simulink model "AutomatedVehicle"  (R2024a)
settings: Solver=FixedStepAuto  StartTime=0.0  StopTime=Tend  FixedStep=Ts  RelTol=1e-3
values from neighbouring files (symbols this model uses):
  ego_v = [4.98933333333 4.97866666667 4.968 4.95733333333 4.94666666667 4.936 4.92533333333 4.91466666667 4.904 4.89333333333 4.88266666667 4.872 ... (5799 elements, 5799x1)]    [SimulationData.mat]    (also in get_Data.m = [ego_v; v])
  ego_x = [2.54994666667 2.59978666667 2.64952 2.69914666667 2.74866666667 2.79808 2.84738666667 2.89658666667 2.94568 2.99466666667 3.04354666667 3.09232 ... (5799 elements, 5799x1)]    [SimulationData.mat]    (also in get_Data.m = [ego_x; egoVehicle.Position(1)])
  ego_y = [-1.65 -1.65 -1.65 -1.65 -1.65 -1.65 -1.65 -1.65 -1.65 -1.65 -1.65 -1.65 ... (5799 elements, 5799x1)]    [SimulationData.mat]    (also in get_Data.m = [ego_y; egoVehicle.Position(2)])
  ego_yaw = [0 0 0 0 0 0 0 0 0 0 0 0 ... (5799 elements, 5799x1)]    [SimulationData.mat]    (also in get_Data.m = [ego_yaw; yaw])
  K1 = Kvec{1}    [Main.m]
  K2 = Kvec{2}    [Main.m]
  K3 = Kvec{3}    [Main.m]
  K4 = Kvec{4}    [Main.m]
  K5 = Kvec{5}    [Main.m]
  K6 = Kvec{6}    [Main.m]
  L = 2.8    [Main.m]
  tau = 0.5    [Main.m]
libraries: simulink x1
settings Model: Creator=mirko  LastModifiedBy=giuco
settings SolverCC: AlgebraicLoopSolver=TrustRegion
settings OptimizationCC: ReuseModelBlockBuffer=off
settings DebuggingCC: UnconnectedInputMsg=warning  UnconnectedOutputMsg=warning  UnconnectedLineMsg=warning
settings ModelReferenceCC: EnableRefExpFcnMdlSchedulingChecks=on
settings SFSimCC: CustomCodeUndefinedFunction=UseInterfaceOnly
settings RTWCC: GPUComputeCapability=3.5

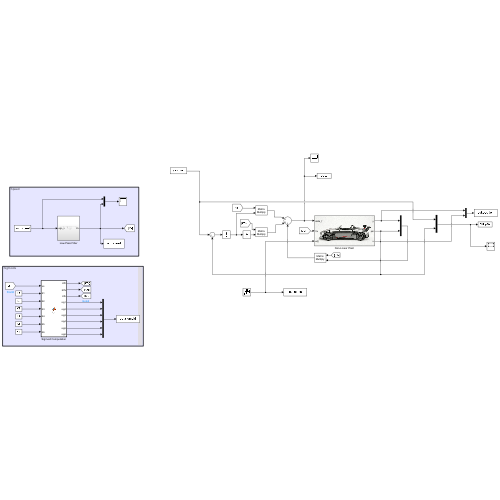
[thumbnail: Simulink's stored preview of the top-level diagram]
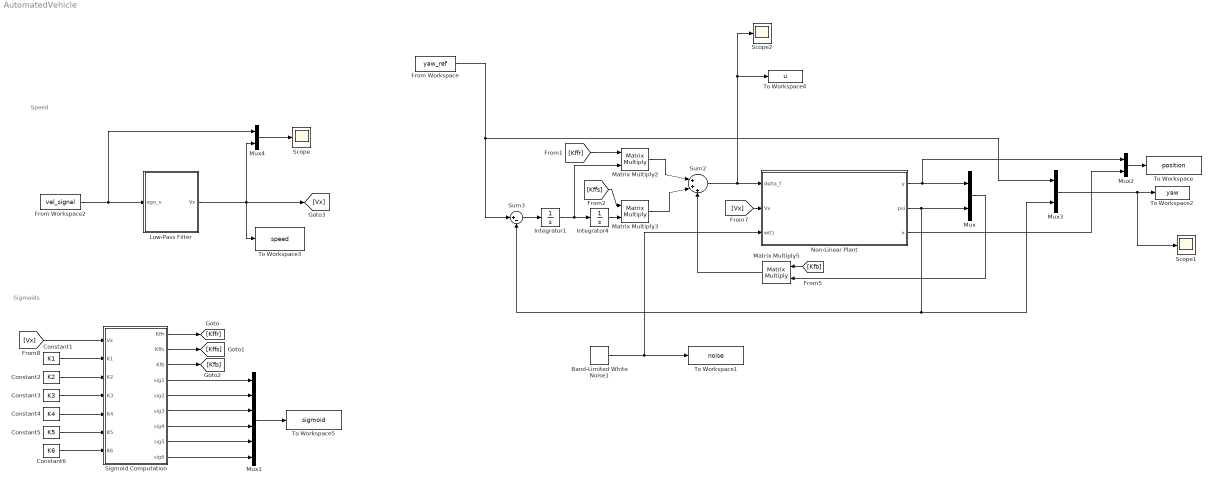
== system AutomatedVehicle ==
  note: Sigmoids
  note: Speed
  Band-Limited White Noise1 : simulink/Sources/Band-Limited White Noise  Cov=[0.001]  Ts=0.1  seed=[23341]
  Constant1 : Constant  Value=K1  VectorParams1D=off
  Constant2 : Constant  Value=K2  VectorParams1D=off
  Constant3 : Constant  Value=K3  VectorParams1D=off
  Constant4 : Constant  Value=K4  VectorParams1D=off
  Constant5 : Constant  Value=K5  VectorParams1D=off
  Constant6 : Constant  Value=K6  VectorParams1D=off
  From Workspace : FromWorkspace  VariableName=yaw_ref
  From Workspace2 : FromWorkspace  VariableName=vel_signal
  Integrator1 : Integrator
  Integrator4 : Integrator
  Low-Pass Filter : Subsystem
  Matrix Multiply2 : Product  Multiplication=Matrix(*)
  Matrix Multiply3 : Product  Multiplication=Matrix(*)
  Matrix Multiply5 : Product  Multiplication=Matrix(*)
  Mux{,2..4} (4 alike) : Mux  Inputs=2
  Mux1 : Mux  Inputs=6
  Non-Linear Plant : Subsystem
      mask Display: image('vehicle.png');
  Scope : Scope
  Scope1 : Scope
  Scope2 : Scope
  Sigmoid Computation : MATLAB Function  TreatAsAtomicUnit=on
  Sum2 : Sum  Inputs=|+++
  Sum3 : Sum  Inputs=|+-
  To Workspace : ToWorkspace  VariableName=position  SaveFormat=Timeseries  SampleTime=-1
  To Workspace1 : ToWorkspace  VariableName=noise  SaveFormat=Timeseries  SampleTime=-1
  To Workspace2 : ToWorkspace  VariableName=yaw  SaveFormat=Timeseries  SampleTime=0.01
  To Workspace3 : ToWorkspace  VariableName=speed  SaveFormat=Timeseries  SampleTime=0.01
  To Workspace4 : ToWorkspace  VariableName=u  SaveFormat=Timeseries  SampleTime=0.01
  To Workspace5 : ToWorkspace  VariableName=sigmoid  SaveFormat=Timeseries  SampleTime=-1
  wires:
  Mux3/1 -> To Workspace2/1, Scope1/1
  Matrix Multiply2/1 -> Sum2/1
  Mux/1 -> Matrix Multiply5/2
  Matrix Multiply3/1 -> Sum2/2
  Matrix Multiply5/1 -> Sum2/3
  Integrator1/1 -> Matrix Multiply2/2, Integrator4/1
  [Vx] -> Non-Linear Plant/2(Vx)
  [Kfb] -> Matrix Multiply5/1
  [Kffs] -> Matrix Multiply3/1
  [Kffr] -> Matrix Multiply2/1
  Sum2/1 -> Non-Linear Plant/1(delta_f), Scope2/1, To Workspace4/1
  From Workspace/1 -> Sum3/1, Mux3/1
  Non-Linear Plant/1(y) -> Mux2/1, Mux/1
  Sum3/1 -> Integrator1/1
  Non-Linear Plant/2(psi) -> Mux/2, Sum3/2, Mux3/2
  Integrator4/1 -> Matrix Multiply3/2
  Non-Linear Plant/3(x) -> Mux2/2
  Sigmoid Computation/1(Kffr) -> [Kffr]
  Constant1/1 -> Sigmoid Computation/2(K1)
  [Vx] -> Sigmoid Computation/1(Vx)
  Sigmoid Computation/2(Kffs) -> [Kffs]
  Sigmoid Computation/3(Kfb) -> [Kfb]
  Low-Pass Filter/1(Vx) -> To Workspace3/1, [Vx], Mux4/2
  From Workspace2/1 -> Low-Pass Filter/1(ego_v), Mux4/1
  Constant2/1 -> Sigmoid Computation/3(K2)
  Constant3/1 -> Sigmoid Computation/4(K3)
  Constant4/1 -> Sigmoid Computation/5(K4)
  Constant5/1 -> Sigmoid Computation/6(K5)
  Constant6/1 -> Sigmoid Computation/7(K6)
  Band-Limited White Noise1/1 -> Non-Linear Plant/3(w(t)), To Workspace1/1
  Sigmoid Computation/4(sig1) -> Mux1/1
  Sigmoid Computation/5(sig2) -> Mux1/2
  Sigmoid Computation/6(sig3) -> Mux1/3
  Sigmoid Computation/7(sig4) -> Mux1/4
  Sigmoid Computation/8(sig5) -> Mux1/5
  Sigmoid Computation/9(sig6) -> Mux1/6
  Mux1/1 -> To Workspace5/1
  Mux2/1 -> To Workspace/1
  Mux4/1 -> Scope/1

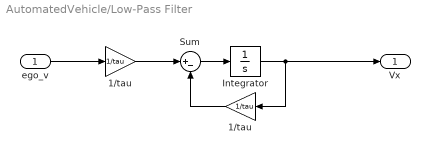
== system AutomatedVehicle/Low-Pass Filter ==
  ego_v : Inport
  1/tau : Gain  Gain=1/tau  SaturateOnIntegerOverflow=on
  "1/tau " : Gain  Gain=1/tau  SaturateOnIntegerOverflow=on
  Integrator : Integrator  InitialCondition=ego_v(1)
  Sum : Sum  Inputs=|+-  SaturateOnIntegerOverflow=on
  Vx : Outport
  wires:
  1/tau/1 -> Sum/1
  Sum/1 -> Integrator/1
  Integrator/1 -> Vx/1, "1/tau "/1
  "1/tau "/1 -> Sum/2
  ego_v/1 -> 1/tau/1

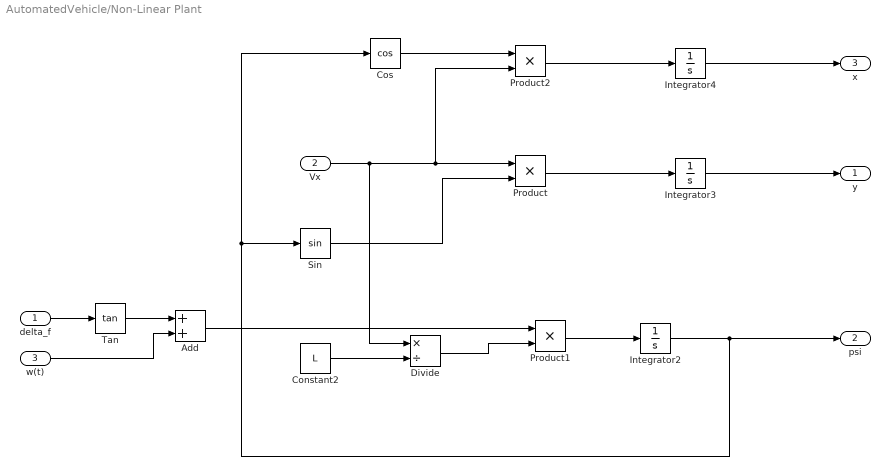
== system AutomatedVehicle/Non-Linear Plant ==
  delta_f : Inport
  Vx : Inport  Port=2
  w(t) : Inport  Port=3
  Add : Sum
  Constant2 : Constant  Value=L
  Cos : Trigonometry  Operator=cos
  Divide : Product  Inputs=*/
  Integrator2 : Integrator  InitialCondition=ego_yaw(1)
  Integrator3 : Integrator  InitialCondition=ego_y(1)
  Integrator4 : Integrator  InitialCondition=ego_x(1)
  Product : Product
  Product1 : Product
  Product2 : Product
  Sin : Trigonometry
  Tan : Trigonometry  Operator=tan
  y : Outport  VectorParamsAs1DForOutWhenUnconnected=off
  psi : Outport  Port=2  VectorParamsAs1DForOutWhenUnconnected=off
  x : Outport  Port=3  VectorParamsAs1DForOutWhenUnconnected=off
  wires:
  Constant2/1 -> Divide/2
  Integrator2/1 -> psi/1, Cos/1, Sin/1
  Divide/1 -> Product1/2
  Product1/1 -> Integrator2/1
  Sin/1 -> Product/2
  Vx/1 -> Product2/2, Product/1, Divide/1
  Cos/1 -> Product2/1
  Integrator3/1 -> y/1
  Product2/1 -> Integrator4/1
  Integrator4/1 -> x/1
  Product/1 -> Integrator3/1
  delta_f/1 -> Tan/1
  w(t)/1 -> Add/2
  Tan/1 -> Add/1
  Add/1 -> Product1/1

== matlab function AutomatedVehicle/Sigmoid Computation ==
  data: Vx input; K1 input; Kffr output; Kffs output; Kfb output; sig1 output; sig2 output; sig3 output; sig4 output; sig5 output; sig6 output; K2 input; K3 input; K4 input; K5 input; K6 input
function [Kffr,Kffs,Kfb,sig1,sig2,sig3,sig4,sig5,sig6] = fcn(Vx,K1,K2,K3,K4,K5,K6)
    bet=10;
    
    sig1=1-1./(1+exp(-bet*(Vx-0.8)));
    sig2=1./(1+exp(-bet*(Vx-0.8)))-1./(1+exp(-bet*(Vx-1.6)));
    sig3=1./(1+exp(-bet*(Vx-1.6)))-1./(1+exp(-bet*(Vx-2.4)));
    sig4=1./(1+exp(-bet*(Vx-2.4)))-1./(1+exp(-bet*(Vx-3.2)));
    sig5=1./(1+exp(-bet*(Vx-3.2)))-1./(1+exp(-bet*(Vx-4.1)));
    sig6=1./(1+exp(-bet*(Vx-4.1)))-1./(1+exp(-bet*(Vx-5)));
    
    % Range1
    %Vertice basso
    kff1_1r = K1(1);
    kff1_1s = K1(2);
    kfb1_1 = K1(3:4);
    %Vertice alto
    kff1_2r = K1(5);
    kff1_2s = K1(6);
    kfb1_2 = K1(7:8);
    
    % Range2
    %Vertice basso
    kff2_1r = K2(1);
    kff2_1s = K2(2);
    kfb2_1 = K2(3:4);
    %Vertice alto
    kff2_2r = K2(5);
    kff2_2s = K2(6);
    kfb2_2 = K2(7:8);
    
    % Range3
    %Vertice basso
    kff3_1r = K3(1);
    kff3_1s = K3(2);
    kfb3_1 = K3(3:4);
    %Vertice alto
    kff3_2r = K3(5);
    kff3_2s = K3(6);
    kfb3_2 = K3(7:8);
    
    % Range4
    %Vertice basso
    kff4_1r = K4(1);
    kff4_1s = K4(2);
    kfb4_1 = K4(3:4);
    %Vertice alto
    kff4_2r = K4(5);
    kff4_2s = K4(6);
    kfb4_2 = K4(7:8);
    
    % Range5
    %Vertice basso
    kff5_1r = K5(1);
    kff5_1s = K5(2);
    kfb5_1 = K5(3:4);
    %Vertice alto
    kff5_2r = K5(5);
    kff5_2s = K5(6);
    kfb5_2 = K5(7:8);
    
    % Range6
    %Vertice basso
    kff6_1r = K6(1);
    kff6_1s = K6(2);
    kfb6_1 = K6(3:4);
    %Vertice alto
    kff6_2r = K6(5);
    kff6_2s = K6(6);
    kfb6_2 = K6(7:8);
    
    % 1: [0, 1] m/s
    p1_1 = (Vx - 0)/(1 - 0); 
    p2_1 = 1 - p1_1;
    
    % 2: [1, 3] m/s
    p1_2 = (Vx - 1)/(3 - 1); 
    p2_2 = 1 - p1_2;
    
    % 3: [3, 6] m/s
    p1_3 = (Vx - 3)/(6 - 3); 
    p2_3 = 1 - p1_3;
    
    % 4: [6, 9] m/s
    p1_4 = (Vx - 6)/(9 - 6); 
    p2_4 = 1 - p1_4;
    
    % 5: [9, 12] m/s
    p1_5 = (Vx - 9)/(12 - 9); 
    p2_5 = 1 - p1_5;
    
    % 6: [12, 14] m/s
    p1_6 = (Vx - 12)/(14 - 12); 
    p2_6 = 1 - p1_6;

    Kffr = sig1*(p1_1*kff1_1r + p2_1*kff1_2r)+...
           sig2*(p1_2*kff2_1r + p2_2*kff2_2r)+...
           sig3*(p1_3*kff3_1r + p2_3*kff3_2r)+...
           sig4*(p1_4*kff4_1r + p2_4*kff4_2r)+...
           sig5*(p1_5*kff5_1r + p2_5*kff5_2r)+...
           sig6*(p1_6*kff6_1r + p2_6*kff6_2r);

    Kffs = sig1*(p1_1*kff1_1s + p2_1*kff1_2s)+...
           sig2*(p1_2*kff2_1s + p2_2*kff2_2s)+...
           sig3*(p1_3*kff3_1s + p2_3*kff3_2s)+...
           sig4*(p1_4*kff4_1s + p2_4*kff4_2s)+...
           sig5*(p1_5*kff5_1s + p2_5*kff5_2s)+...
           sig6*(p1_6*kff6_1s + p2_6*kff6_2s);

    Kfb = sig1*(p1_1*kfb1_1 + p2_1*kfb1_2)+...
          sig2*(p1_2*kfb2_1 + p2_2*kfb2_2)+...
          sig3*(p1_3*kfb3_1 + p2_3*kfb3_2)+...
          sig4*(p1_4*kfb4_1 + p2_4*kfb4_2)+...
          sig5*(p1_5*kfb5_1 + p2_5*kfb5_2)+...
          sig6*(p1_6*kfb6_1 + p2_6*kfb6_2);

end
